simulink model "Model"  (R2018b)
settings: Solver=ode4  StartTime=0.0  StopTime=100.0  FixedStep=0.01  RelTol=1e-3  EnableMultiTasking=on
libraries: simulink x1
settings Model: Creator=lpa2  LastModifiedBy=Kasia
settings SolverCC: AutoInsertRateTranBlk=on
settings DataIOCC: LimitDataPoints=on
settings OptimizationCC: LifeSpan=inf
settings DebuggingCC: AllowSymbolicDim=off  SFUnexpectedBacktrackingDiag=warning  SFNoUnconditionalDefaultTransitionDiag=warning  SFExecutionAtInitializationDiag=none
settings ModelReferenceCC: PropagateSignalLabelsOutOfModel=off
settings SFSimCC: SimUseLocalCustomCode=off
settings RTWCC: RTWUseLocalCustomCode=off
settings CodeAppCC: StateflowObjectComments=on
settings GRTTargetCC: TargetLangStandard=C89/C90 (ANSI)
settings ConfigComp: CovMetricSettings=dw  CovHtmlReporting=on  CovSaveCumulativeToWorkspaceVar=on  CovSaveSingleToWorkspaceVar=on  CovExternalEMLEnable=off

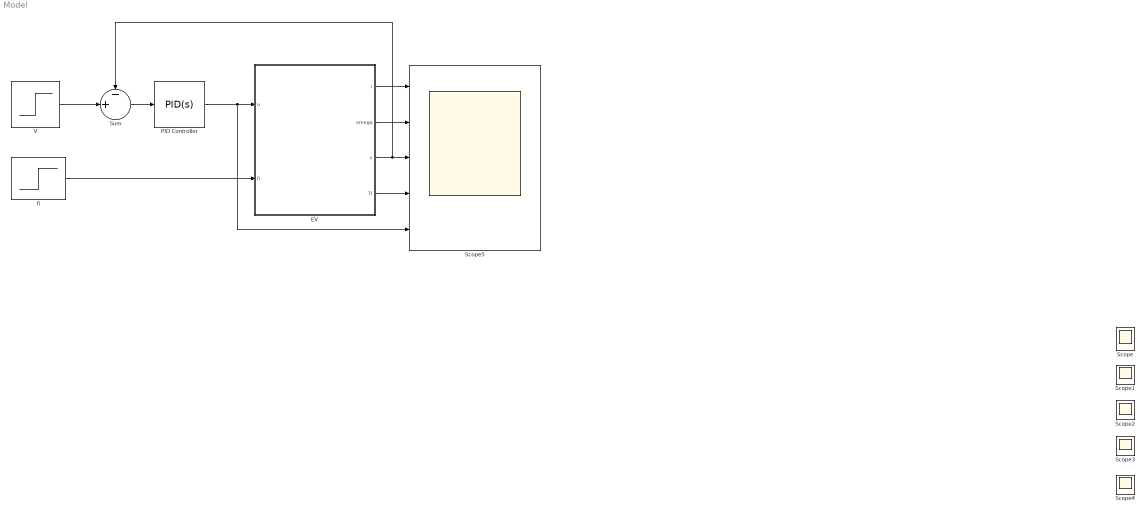
== system Model ==
  EV : Subsystem
  PID Controller : simulink/Continuous/PID Controller  Controller=PID  Form=Parallel  TimeDomain=Continuous-time  SampleTime=-1  IntegratorMethod=Forward Euler  FilterMethod=Forward Euler  ControllerParametersSource=internal  P=4.28638411324933  I=0.581025934902661  D=-2.03238817276156  UseFilter=on  N=0.205433389361967  TunerSelectOption=Transfer Function Based (PID Tuner App)  InitialConditionSource=internal  InitialConditionForIntegrator=0  InitialConditionForFilter=0  DifferentiatorICPrevScaledInput=0  ExternalReset=none  TrackingMode=off  Kt=1  LimitOutput=on  UpperSaturationLimit=48  LowerSaturationLimit=0  LinearizeAsGain=on  AntiWindupMode=clamping  Kb=1  POutMin=[]  POutMax=[]  IOutMin=[]  IOutMax=[]  DOutMin=[]  DOutMax=[]  NOutMin=[]  NOutMax=[]  SumOutMin=[]  SumOutMax=[]  SaturationOutMin=[]  SaturationOutMax=[]  PParamMin=[]  PParamMax=[]  IParamMin=[]  IParamMax=[]  DParamMin=[]  DParamMax=[]  NParamMin=[]  NParamMax=[]  KbParamMin=[]  KbParamMax=[]  KtParamMin=[]  KtParamMax=[]  KbOutMin=[]  KbOutMax=[]  KtOutMin=[]  KtOutMax=[]  IntegratorOutMin=[]  IntegratorOutMax=[]  FilterOutMin=[]  FilterOutMax=[]  SumI1OutMin=[]  SumI1OutMax=[]  SumI2OutMin=[]  SumI2OutMax=[]  SumI3OutMin=[]  SumI3OutMax=[]  SumI4OutMin=[]  SumI4OutMax=[]  SumDOutMin=[]  SumDOutMax=[]  DifferentiatorOutMin=[]  DifferentiatorOutMax=[]  FilterDiffOutCoefMin=[]  FilterDiffOutCoefMax=[]  ReciprocalOutMin=[]  ReciprocalOutMax=[]  SumDenOutMin=[]  SumDenOutMax=[]  SumNumOutMin=[]  SumNumOutMax=[]  DivideOutMin=[]  DivideOutMax=[]  IntegratorContinuousStateAttributes=''  IntegratorStateMustResolveToSignalObject=off  IntegratorRTWStateStorageClass=Auto  FilterContinuousStateAttributes=''  FilterStateMustResolveToSignalObject=off  FilterRTWStateStorageClass=Auto  ParallelPVariant=InternalParameters  IdealPVariant=Disabled  IVariant=InternalParameters  DVariant=InternalParameters  IntegratorVariant=Continuous  SatVariant=Enabled  AWVariant=ContClampingParallel  PCopyVariant=Disabled  TRVariant=Disabled  FdbkBlocksVariant=Forward  IdealPFdbkVariant=Disabled  SatFdbkVariant=Disabled  DerivativeFilterVariant=ContFilter  NVariant=InternalParameters  NCopyVariant=Disabled  FilterICVariant=InternalICsFilter  IntegratorICVariant=InternalICs  ExternalResetVariant=Disabled  TRSumVariant=Passthrough  SumFdbkVariant=Disabled  SumVariant=Sum_PID
  Scope{,1..4} (5 alike) : Scope
  Scope5 : Scope  NumInputPorts=5
  Sum : Sum  Inputs=-+|
  V : Step  After=10*1000/3600  SampleTime=1
  fi : Step  Time=50  After=3*pi/180  SampleTime=1
  wires:
  V/1 -> Sum/2
  Sum/1 -> PID Controller/1
  PID Controller/1 -> Scope5/5, EV/1(u)
  EV/4(TI) -> Scope5/4
  EV/2("omega ") -> Scope5/2
  EV/1(I) -> Scope5/1
  EV/3(v) -> Sum/1, Scope5/3
  fi/1 -> EV/2(fi)
  ? -> Scope3/1
  ? -> Scope/1
  ? -> Scope1/1
  ? -> Scope2/1
  ? -> Scope4/1

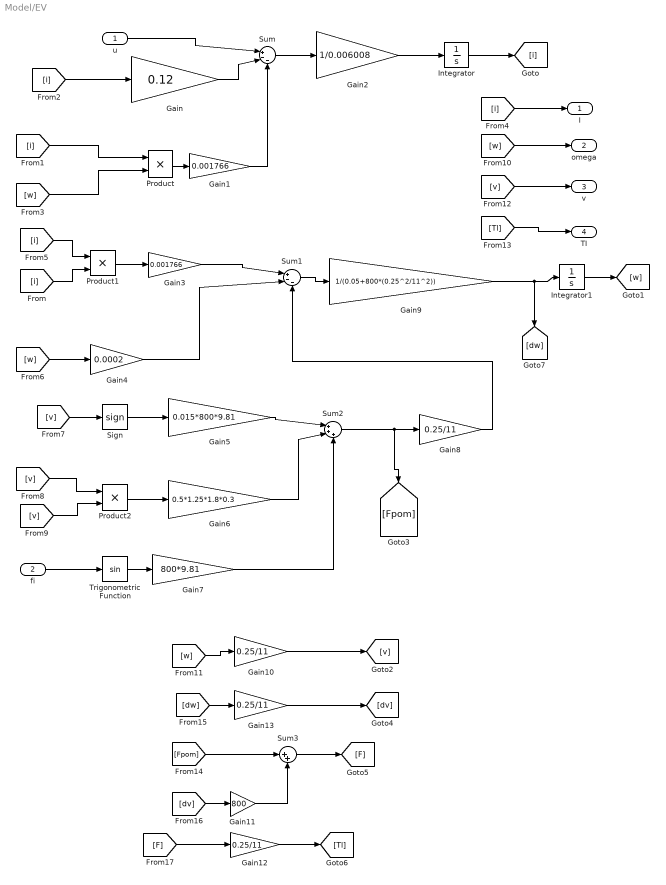
== system Model/EV ==
  u : Inport
  fi : Inport  Port=2
  Gain : Gain  Gain=0.12
  Gain1 : Gain  Gain=0.001766
  Gain{8,10,12..13} (4 alike) : Gain  Gain=0.25/11
  Gain11 : Gain  Gain=800
  Gain2 : Gain  Gain=1/0.006008
  Gain3 : Gain  Gain=0.001766
  Gain4 : Gain  Gain=0.0002
  Gain5 : Gain  Gain=0.015*800*9.81
  Gain6 : Gain  Gain=0.5*1.25*1.8*0.3
  Gain7 : Gain  Gain=800*9.81
  Gain9 : Gain  Gain=1/(0.05+800*(0.25^2/11^2))
  Integrator : Integrator  LimitOutput=on  UpperSaturationLimit=250
  Integrator1 : Integrator
  Product : Product
  Product1 : Product
  Product2 : Product
  Sign : Signum
  Sum : Sum  Inputs=|+--
  Sum1 : Sum  Inputs=|+--
  Sum2 : Sum  Inputs=|+++
  Sum3 : Sum  Inputs=|++
  Trigonometric Function : Trigonometry
  I : Outport
  "omega " : Outport  Port=2
  v : Outport  Port=3
  TI : Outport  Port=4
  wires:
  [i] -> Product/1
  Sum/1 -> Gain2/1
  u/1 -> Sum/1
  Gain/1 -> Sum/2
  Integrator/1 -> [i]
  Product/1 -> Gain1/1
  [w] -> Product/2
  [i] -> Gain/1
  Gain2/1 -> Integrator/1
  [i] -> I/1
  [i] -> Product1/1
  [i] -> Product1/2
  Product1/1 -> Gain3/1
  Gain3/1 -> Sum1/1
  [w] -> Gain4/1
  Gain4/1 -> Sum1/2
  [v] -> Sign/1
  Sign/1 -> Gain5/1
  Gain5/1 -> Sum2/1
  [v] -> Product2/1
  [v] -> Product2/2
  Product2/1 -> Gain6/1
  Gain6/1 -> Sum2/2
  Trigonometric Function/1 -> Gain7/1
  Gain7/1 -> Sum2/3
  Sum2/1 -> Gain8/1, [Fpom]
  Gain8/1 -> Sum1/3
  Sum1/1 -> Gain9/1
  Gain9/1 -> Integrator1/1, [dw]
  Integrator1/1 -> [w]
  [w] -> Gain10/1
  Gain10/1 -> [v]
  fi/1 -> Trigonometric Function/1
  [w] -> "omega "/1
  [v] -> v/1
  [dv] -> Gain11/1
  Gain11/1 -> Sum3/2
  [Fpom] -> Sum3/1
  Sum3/1 -> [F]
  [F] -> Gain12/1
  Gain12/1 -> [Tl]
  [Tl] -> TI/1
  [dw] -> Gain13/1
  Gain13/1 -> [dv]
  Gain1/1 -> Sum/3
